simulink model "Demo_SteerableHeadlights_cs"  (Simulink 7.6)
settings: Solver=FixedStepDiscrete  SolverMode=SingleTasking  StartTime=0.0  StopTime=45  FixedStep=1/20  RelTol=1e-3
model workspace (MAT data in the model file):
  mbox_table : struct (value not decoded)
  model_closed = 0
  sim_status = 0
PreLoadFcn:
  | check_NUTS_defined;
  | 
  | assignin('base',['model_closed_' bdroot],false);
InitFcn:
  | PreScanExperimentInitFcn(bdroot)
StopFcn:
  | PreScanExperimentStopFcn(bdroot)
undefined symbols (not defined in the file or in its folder): DiscIntNeverNeededParam, x_ini_VRML, y_ini_VRML, z_ini_VRML
libraries: PreScanSimulinkLibrary x9, simulink_extras x6, simulink x4, PreScanUsefulBlocks x2
(part 1 of 4)
CloseFcn:
  | evalin('base',['clear model_closed_' bdroot]);
settings Model: Creator=PRESCAN  LastModifiedBy=buildbot
settings OptimizationCC: InitFltsAndDblsToZero=on
settings DebuggingCC: SaveWithParameterizedLinksMsg=none  SignalResolutionControl=TryResolveAllWithWarning  MultiTaskDSMMsg=warning  MultiTaskCondExecSysMsg=none
settings SFSimCC: SimParseCustomCode=off
settings RTWCC: IncludeERTFirstTime=on
settings GRTTargetCC: TargetFcnLib=ansi_tfl_tmw.mat

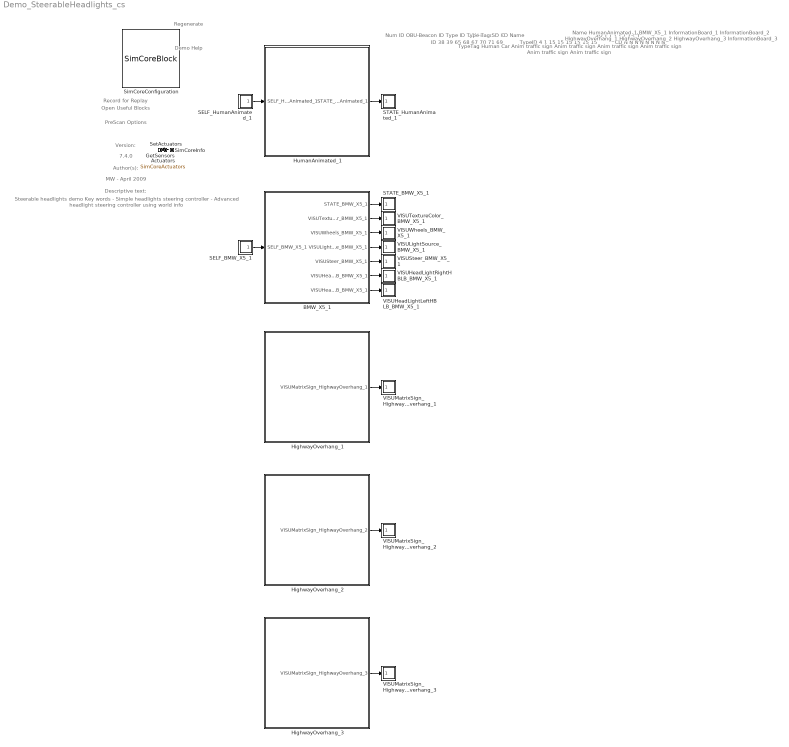
== system Demo_SteerableHeadlights_cs ==
  note: Demo Help
  note: Regenerate
  note: Record for Replay
  note: Open Useful Blocks
  note: PreScan Options
  note: Version:
  note: 7.4.0
  note: Author(s):
  note: MW - April 2009
  note: Descriptive text:
  note: Steerable headlights demo
      |
      | Key words
      | - Simple headlights steering
      | controller
      | - Advanced headlight steering
      | controller using world info
  note: ID
      |
      | 38
      | 39
      | 65
      | 68
      | 67
      | 70
      | 71
      | 69
  note: OBU-Beacon ID
  note: TypeID
      |
      | 4
      | 1
      | 15
      | 15
      | 15
      | 15
      | 15
      | 15
  note: TypeTag
      |
      | Human
      | Car
      | Anim traffic sign
      | Anim traffic sign
      | Anim traffic sign
      | Anim traffic sign
      | Anim traffic sign
      | Anim traffic sign
  note: SD
      |
      | Y
      | Y
      | Y
      | Y
      | Y
      | Y
      | Y
      | Y
  note: CD
      |
      | N
      | N
      | N
      | N
      | N
      | N
      | N
      | N
  note: Name
      |
      | HumanAnimated_1
      | BMW_X5_1
      | InformationBoard_1
      | InformationBoard_2
      | HighwayOverhang_1
      | HighwayOverhang_2
      | HighwayOverhang_3
      | InformationBoard_3
  note: Num ID OBU-Beacon ID Type ID Type Tag SD CD Name
  Actuators : DataStoreMemory  Tag=Actuators  DataStoreName=SimCoreActuators  InitialValue=zeros(288,1)
      settings: DeleteFcn=PreScanBlockDeleteFcn;
  BMW_X5_1 : Subsystem  Tag=WorldObjectSubSystem  InitFcn=UniqueId = '67';
      mask Display: image(imread('BMW_X5.jpg'));color('white');text(0,0,' ID=39\n')
  GetSensors : Subsystem  Tag=GetSensors  Priority=2  mask(PreScan Simulation Core Block){NrOfSensors=16, TimeStep=1/20}
      mask prompts: NrOfSensors "Number of sensor values"; TimeStep "Timestep [s]"
      mask help:
      | Please do not remove this block from the PreScan compilation sheet,
      | as it contains essential configuration parameters for a PreScan simulation.
      settings: DeleteFcn=PreScanBlockDeleteFcn;
  HighwayOverhang_1 : Subsystem  Tag=WorldObjectSubSystem  InitFcn=UniqueId = '104';
      mask Display: image(imread('HighwayOverhang.jpg'));color('white');text(0,0,' ID=67\n')
  HighwayOverhang_2 : Subsystem  Tag=WorldObjectSubSystem  InitFcn=UniqueId = '106';
      mask Display: image(imread('HighwayOverhang.jpg'));color('white');text(0,0,' ID=70\n')
  HighwayOverhang_3 : Subsystem  Tag=WorldObjectSubSystem  InitFcn=UniqueId = '108';
      mask Display: image(imread('HighwayOverhang.jpg'));color('white');text(0,0,' ID=71\n')
  HumanAnimated_1 : Subsystem  Tag=WorldObjectSubSystem  InitFcn=UniqueId = '63';
      mask Display: image(imread('HumanAnimated.jpg'));color('white');text(0,0,' ID=38\n')
  SELF_BMW_X5_1 : Subsystem  Tag=SELF  Priority=3  mask(PreScan Source Block: SELF){PortName=SELF_BMW_X5_1, PortIndex=8, PortWidth=8, TimeStep=1/20}
      mask prompts: PortName "Auto-Assigned: Port Name [-]"; PortIndex "Auto-Assigned: Port Index [-]"; PortWidth "Auto-Assigned: Port Dimensions"; TimeStep "Auto-Assigned: Upload Period [s]"
      mask help:
      | The SELF port shows (state) information of the actor itself. The outputs are position in the experiment's axis system and the GPS coordinates, and the object's absolute velocity and compass heading.
      |
      | For more information, please click Help.
      settings: DeleteFcn=PreScanBlockDeleteFcn;
      mask Help: eval('openHelp(462)')
      mask Display: image(imread('GPS.png'))
  SELF_HumanAnimated_1 : Subsystem  Tag=SELF  Priority=3  mask(PreScan Source Block: SELF){PortName=SELF_HumanAnimated_1, PortIndex=0, PortWidth=8, TimeStep=1/20}
      mask prompts: PortName "Auto-Assigned: Port Name [-]"; PortIndex "Auto-Assigned: Port Index [-]"; PortWidth "Auto-Assigned: Port Dimensions"; TimeStep "Auto-Assigned: Upload Period [s]"
      mask help:
      | The SELF port shows (state) information of the actor itself. The outputs are position in the experiment's axis system and the GPS coordinates, and the object's absolute velocity and compass heading.
      |
      | For more information, please click Help.
      settings: DeleteFcn=PreScanBlockDeleteFcn;
      mask Help: eval('openHelp(462)')
      mask Display: image(imread('GPS.png'))
  STATE_BMW_X5_1 : Subsystem  Tag=State  Priority=0  mask(PreScan Sink Block: State){x0=0.147277832, y0=0.07363796, z0=0.69, Roll0=0, Pitch0=0, Yaw0=0, TimeStep=1/20}
      mask prompts: x0 "Ini x-position VEHICLE wrt GLOBAL axis system [m]"; y0 "Ini y-position VEHICLE wrt GLOBAL axis system [m]"; z0 "Ini z-position VEHICLE wrt GLOBAL axis system [m]"; Roll0 "Ini roll-angle BODY wrt VEHICLE axis system [deg]"; Pitch0 "Ini pitch-angle BODY wrt VEHICLE axis system [deg]"; Yaw0 "Ini yaw-angle VEHICLE wrt GLOBAL axis system [deg]"; TimeStep "Time Step [s]"
      mask help:
      | The Actor State contains a vector signal of size (9x1), containing the following signals:
      |
      | -  Position                  (x,y,z)                                     [m]
      | -  Velocity                  (vx,vy,vz)                               [m/s]
      | -  Angles                    (Roll, Pitch, Yaw)                   [rad]
      |
      | The Actor state is defined in the global axis system.
      | The state is superponed on the Initial position defined in the GUI.
      |
      | For more information, please click Help.
      settings: DeleteFcn=PreScanBlockDeleteFcn;
      mask Help: eval('openHelp(222)')
      mask Display: image(imread('State.png'))
  STATE_HumanAnimated_1 : Subsystem  Tag=StateAnim  Priority=0  mask(PreScan Sink Block: StateAnim){x0=294.188263, y0=-30, z0=0, Roll0=0, Pitch0=0, Yaw0=102.59381900000001, TimeStep=1/20, MWS=1.95}
      mask prompts: x0 "Ini x-position VEHICLE wrt GLOBAL axis system [m]"; y0 "Ini y-position VEHICLE wrt GLOBAL axis system [m]"; z0 "Ini z-position VEHICLE wrt GLOBAL axis system [m]"; Roll0 "Ini roll-angle BODY wrt GLOBAL axis system [rad]"; Pitch0 "Ini pitch-angle BODY wrt GLOBAL axis system [rad]"; Yaw0 "Ini yaw-angle BODY wrt GLOBAL axis system [rad]"; TimeStep "Time Step [s]"; MWS "Max Walking Speed [m/s]"
      mask help:
      | The Actor State contains a vector signal of size (9x1), containing the following signals:
      |
      | -  Position                  (x,y,z)                                     [m]
      | -  Velocity                  (vx,vy,vz)                               [m/s]
      | -  Angles                    (Roll, Pitch, Yaw)                   [rad]
      |
      | The Actor state is defined in the global axis system.
      | The state is superponed on the Initial position defined in the GUI.
      |
      | For more information, please click Help.
      settings: DeleteFcn=PreScanBlockDeleteFcn;
      mask Help: eval('openHelp(222)')
      mask Display: image(imread('StateAnim.png'))
  SetActuators : Subsystem  Tag=SetActuators  Priority=1  mask(PreScan Simulation Core Block){TimeStep=1/20, NrOfActuators=288}
      mask prompts: TimeStep "Timestep [s]"; NrOfActuators "Number of actuator values"
      mask help:
      | Please do not remove this block from the PreScan compilation sheet,
      | as it contains essential configuration parameters for a PreScan simulation.
      settings: DeleteFcn=PreScanBlockDeleteFcn;
  SimCoreConfiguration : M-S-Function  Tag=SimCoreConfiguration  Description=D0CC6153B97817DA1051E6984CAAAF7B53F59DDD33C61524121AC7332DD66955  FunctionName=SimCoreBlock  Parameters=ExperimentXML PortsXML SimulationCore HostName CheckStart EnableLog RfR EnableGPUAccel ShowComputationTime  mask(PreScan Simulation Core Configurator){SimulationCore=NUTS, HostName=0, CheckStart=0, prescanversion='7.4.0', EnableLog=off, RfR=0, EnableGPUAccel=off, ShowComputationTime=off}
      mask prompts: SimulationCore "Simulation Core"; HostName "Simulation Host"; CheckStart "Show START Dialog"; prescanversion "PreScan Version"; EnableLog "Create TA Log"; RfR "Record for Replay"; EnableGPUAccel "Enable GPU Acceleration"; ShowComputationTime "Show ComputationTime Scope"
      mask help:
      | Please do not remove this block from the PreScan compilation sheet,
      | as it contains essential configuration parameter for a PreScan simulation.
      mask init:
      | model = bdroot;
      | ExperimentXML = [model(1:end-3) '.pex'];
      | PortsXML = [model '_ports.pcd'];
      settings: DeleteFcn=PreScanBlockDeleteFcn;  ModelCloseFcn=assignin('base',['model_closed_' bdroot],true);
      mask Help: eval('openHelp(812)')
      mask Display: image(imread('prescanlogo.ico'))
  SimCoreInfo : Subsystem  Tag=SimCoreInfo
  VISUHeadLightLeftHBLB_BMW_X5_1 : Subsystem  Tag=VisuLights  Priority=0
      settings: DeleteFcn=PreScanBlockDeleteFcn;
      mask Type: PreScan Sink Block: VisuLights
      mask Description:
      | The VisuLights block provides a way to animate the active lights of a vehicle with possibilities to adapt the:
      | - Intensity [-]
      | - Position (x,y,z) [m]
      | - Orientation (Roll, Pitch, Yaw) [deg]
      | - Color (RGB) [-]
      | - TextureResourceID [-]
      | 
      | For more information, please click Help.
      mask Help: eval('openHelp(231)')
      mask Display: image(imread('HeadLight.png'))
  VISUHeadLightRightHBLB_BMW_X5_1 : Subsystem  Tag=VisuLights  Priority=0
      settings: DeleteFcn=PreScanBlockDeleteFcn;
      mask Type: PreScan Sink Block: VisuLights
      mask Description:
      | The VisuLights block provides a way to animate the active lights of a vehicle with possibilities to adapt the:
      | - Intensity [-]
      | - Position (x,y,z) [m]
      | - Orientation (Roll, Pitch, Yaw) [deg]
      | - Color (RGB) [-]
      | - TextureResourceID [-]
      | 
      | For more information, please click Help.
      mask Help: eval('openHelp(231)')
      mask Display: image(imread('HeadLight.png'))
  VISULightSource_BMW_X5_1 : Subsystem  Tag=VisuLightSource  Priority=0
      settings: DeleteFcn=PreScanBlockDeleteFcn;
      mask Type: PreScan Sink Block: VisuLightSource
      mask Description:
      | The VisuLightSource block provides a way to animate Light Sources of the indicator, braking, fog and main lights of a vehicle.
      | 
      | For more information, please click Help.
      mask Help: eval('openHelp(223)')
      mask Display: image(imread('RearLight.png'))
  VISUMatrixSign_HighwayOverhang_1 : Subsystem  Tag=VisuMatrixSign  Priority=0
      settings: DeleteFcn=PreScanBlockDeleteFcn;
      mask Type: PreScan Sink Block: VisuMatrixSign
      mask Description:
      | The VisuMatrixSign block provides a way to adapt the texture of the plates connected to an overhang, based on Resource IDs of the texture files.
      | 
      | For more information, please click Help.
      mask Help: eval('openHelp()')
      mask Display: image(imread('HighwaySpeedMatrix.png'))
  VISUMatrixSign_HighwayOverhang_2 : Subsystem  Tag=VisuMatrixSign  Priority=0
      settings: DeleteFcn=PreScanBlockDeleteFcn;
      mask Type: PreScan Sink Block: VisuMatrixSign
      mask Description:
      | The VisuMatrixSign block provides a way to adapt the texture of the plates connected to an overhang, based on Resource IDs of the texture files.
      | 
      | For more information, please click Help.
      mask Help: eval('openHelp()')
      mask Display: image(imread('HighwaySpeedMatrix.png'))
  VISUMatrixSign_HighwayOverhang_3 : Subsystem  Tag=VisuMatrixSign  Priority=0
      settings: DeleteFcn=PreScanBlockDeleteFcn;
      mask Type: PreScan Sink Block: VisuMatrixSign
      mask Description:
      | The VisuMatrixSign block provides a way to adapt the texture of the plates connected to an overhang, based on Resource IDs of the texture files.
      | 
      | For more information, please click Help.
      mask Help: eval('openHelp()')
      mask Display: image(imread('HighwaySpeedMatrix.png'))
  VISUSteer_BMW_X5_1 : Subsystem  Tag=VisuSteer  Priority=0
      settings: DeleteFcn=PreScanBlockDeleteFcn;
      mask Type: PreScan Sink Block: VisuSteer
      mask Description:
      | The VisuSteer block provides a way to adapt the orientation of the steering column and steering wheel of a vehicle.
      | 
      | For more information, please click Help.
      mask Help: eval('openHelp(223)')
      mask Display: image(imread('steeringwheel.png'))
  VISUTextureColor_BMW_X5_1 : Subsystem  Tag=VisuTextureColor  Priority=0
      settings: DeleteFcn=PreScanBlockDeleteFcn;
      mask Type: PreScan Sink Block: VisuTextureColor
      mask Description:
      | The Texture Color block provides a way to adapt the color of a vehicle.
      | 
      | For more information, please click Help.
      mask Help: eval('openHelp(230)')
      mask Display: image(imread('TextureColor.png'))
  VISUWheels_BMW_X5_1 : Subsystem  Tag=VisuWheels  Priority=0
      settings: DeleteFcn=PreScanBlockDeleteFcn;
      mask Type: PreScan Sink Block: VisuWheels
      mask Description:
      | The VisuWheels block provides a way to animate the wheels of a vehicle, with steering, rotation (because of velocity) and z-displacement.
      | 
      | For more information, please click Help.
      mask Help: eval('openHelp(223)')
      mask Display: image(imread('wheel.png'))
  wires:
  HumanAnimated_1/1(STATE_HumanAnimated_1) -> STATE_HumanAnimated_1/1(State)
  SELF_HumanAnimated_1/1(U) -> HumanAnimated_1/1(SELF_HumanAnimated_1)
  BMW_X5_1/1(STATE_BMW_X5_1) -> STATE_BMW_X5_1/1(State)
  SELF_BMW_X5_1/1(U) -> BMW_X5_1/1(SELF_BMW_X5_1)
  BMW_X5_1/2(VISUTextureColor_BMW_X5_1) -> VISUTextureColor_BMW_X5_1/1(TextureColor)
  BMW_X5_1/3(VISUWheels_BMW_X5_1) -> VISUWheels_BMW_X5_1/1(Wheels)
  BMW_X5_1/4(VISULightSource_BMW_X5_1) -> VISULightSource_BMW_X5_1/1(Lights)
  BMW_X5_1/5(VISUSteer_BMW_X5_1) -> VISUSteer_BMW_X5_1/1(Steer)
  BMW_X5_1/6(VISUHeadLightRightHBLB_BMW_X5_1) -> VISUHeadLightRightHBLB_BMW_X5_1/1(Lights)
  BMW_X5_1/7(VISUHeadLightLeftHBLB_BMW_X5_1) -> VISUHeadLightLeftHBLB_BMW_X5_1/1(Lights)
  HighwayOverhang_1/1(VISUMatrixSign_HighwayOverhang_1) -> VISUMatrixSign_HighwayOverhang_1/1(MatrixSigns)
  HighwayOverhang_2/1(VISUMatrixSign_HighwayOverhang_2) -> VISUMatrixSign_HighwayOverhang_2/1(MatrixSigns)
  HighwayOverhang_3/1(VISUMatrixSign_HighwayOverhang_3) -> VISUMatrixSign_HighwayOverhang_3/1(MatrixSigns)
  SetActuators/1(dummy) -> GetSensors/1(dummy)

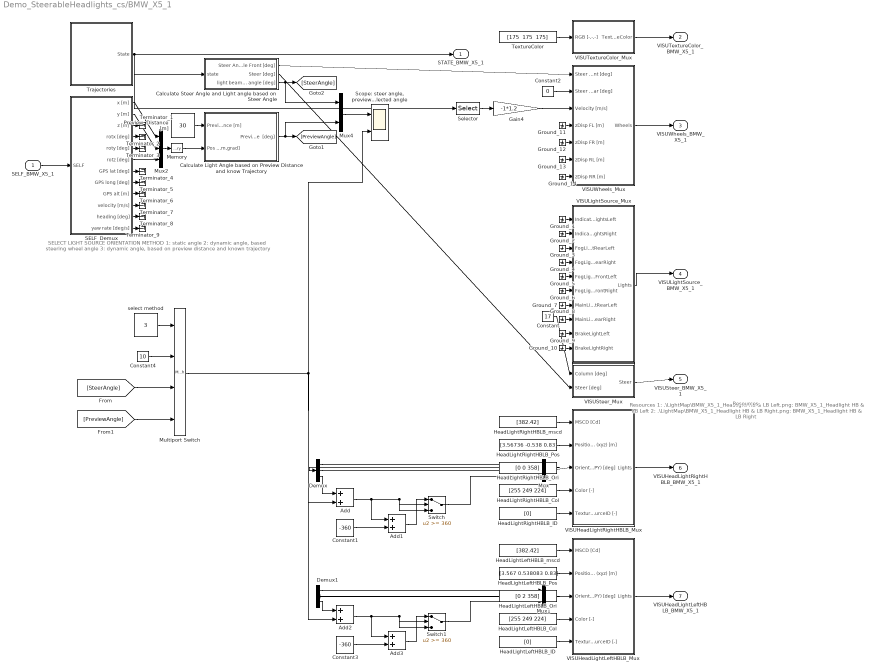
== system Demo_SteerableHeadlights_cs/BMW_X5_1 ==
  note: SELECT LIGHT SOURCE ORIENTATION METHOD
      | 1: static angle
      | 2: dynamic angle, based steering wheel angle
      | 3: dynamic angle, based on preview distance
      |     and known trajectory
  note: Resources
      |
      | 1: .\LightMap\BMW_X5_1_Headlight HB & LB Left.png: BMW_X5_1_Headlight HB & LB Left
      | 2: .\LightMap\BMW_X5_1_Headlight HB & LB Right.png: BMW_X5_1_Headlight HB & LB Right
  note: Resources
  SELF_BMW_X5_1 : Inport  Tag=SELFInport
  Add{,1..3} (4 alike) : Sum
  Calculate Light Angle based on Preview Distance and know Trajectory : Subsystem  mask{FileName=PathFollowerSva_1_Synced.mat, TrajOffset=[0 0 0]}
      mask prompts: FileName "Trajectory Name"; TrajOffset "Trajectory Initial Offset x,y,yawangle [m,m,rad]"
      mask init:
      | load(['trajectories/',FileName])
      | traject=trajectory';
      | 
      | 
      | Traj_x=(traject(:,2)*cos(TrajOffset(3))-traject(:,3)*sin(TrajOffset(3)))+TrajOffset(1);
      | Traj_y=(traject(:,2)*sin(TrajOffset(3))+traject(:,3)*cos(TrajOffset(3)))+TrajOffset(2);
  Calculate Steer Angle and Light angle based on  Steer Angle : Subsystem
  Constant : Constant  Value=17
  Constant1 : Constant  Value=-360
  Constant2 : Constant  Value=0
  Constant3 : Constant  Value=-360
  Constant4 : Constant  Value=10
  Demux : Demux  Outputs=3
  Demux1 : Demux  Outputs=3
  Gain4 : Gain  Gain=-1*1.2
  Ground_{1..14} (14 alike) : Ground
  HeadLightLeftHBLB_Col : Constant  Tag=VisuLightConst  Value=[255 249 224]
  HeadLightLeftHBLB_ID : Constant  Tag=VisuLightConst  Value=[0]
  HeadLightLeftHBLB_Ori : Constant  Tag=VisuLightConst  Value=[0 2 358]
  HeadLightLeftHBLB_Pos : Constant  Tag=VisuLightConst  Value=[3.567 0.538083 0.83]
  HeadLightLeftHBLB_mscd : Constant  Tag=VisuLightConst  Value=[382.42]
  HeadLightRightHBLB_Col : Constant  Tag=VisuLightConst  Value=[255 249 224]
  HeadLightRightHBLB_ID : Constant  Tag=VisuLightConst  Value=[0]
  HeadLightRightHBLB_Ori : Constant  Tag=VisuLightConst  Value=[0 0 358]
  HeadLightRightHBLB_Pos : Constant  Tag=VisuLightConst  Value=[3.56736 -0.538 0.83]
  HeadLightRightHBLB_mscd : Constant  Tag=VisuLightConst  Value=[382.42]
  Memory : Memory
  Multiport Switch : MultiPortSwitch  zeroidx=off
  Mux : Mux  Inputs=3
  Mux1 : Mux  Inputs=3
  Mux2 : Mux  Inputs=3
  Mux4 : Mux  Inputs=2
  Preview  Distance [m] : Constant  Value=30
  SELF_Demux : Subsystem  Tag=DemuxSELF
      settings: DeleteFcn=PreScanBlockDeleteFcn;
      mask Type: PreScan Demux Block:
      mask Display:
      | port_label('output',1,'x [m]')
      | port_label('output',2,'y [m]')
      | port_label('output',3,'z [m]','texmode','on')
      | port_label('output',4,'Rotx [deg]','texmode','on')
      | port_label('output',5,'Roty [deg]','texmode','on')
      | port_label('output',6,'Rotz [deg]','texmode','on')
      | port_label('output',7,'GPS lat [deg]','texmode','on')
      | port_label('output',8,'GPS long [deg]','texmode','on')
      | port_label('output',9,'GPS alt [m]','texmode','on')
      | port_label('output',10,'Velocity [m/s]')
      | port_label('output',11,'Heading [deg]')
      | port_label('output',12,'Yaw rate [deg/s]')
  "Scope: steer angle, preview angle, selected angle" : Scope  NumInputPorts=2
      settings: TimeRange=45  YMin=-50~-40  YMax=60~45  SaveName=ScopeData2
  Selector : Selector  InputPortWidth=9  IndexOptions=Index vector (dialog)  Indices=4  OutputSizes=1
  Switch : Switch  Threshold=360
  Switch1 : Switch  Threshold=360
  Terminator_{1..9} (9 alike) : Terminator
  TextureColor : Constant  Tag=TextureColor  Value="[175  175  175]"
  Trajectories : Subsystem  Tag=Trajectories
      settings: DeleteFcn=PreScanBlockDeleteFcn;
      mask Display: image(imread('Trajectory.png'));
  VISUHeadLightLeftHBLB_Mux : Subsystem  Tag=MuxLights
      settings: DeleteFcn=PreScanBlockDeleteFcn;
      mask Type: PreScan Mux Block:
  VISUHeadLightRightHBLB_Mux : Subsystem  Tag=MuxLights
      settings: DeleteFcn=PreScanBlockDeleteFcn;
      mask Type: PreScan Mux Block:
  VISULightSource_Mux : Subsystem  Tag=MuxLightSource
      settings: DeleteFcn=PreScanBlockDeleteFcn;
      mask Type: PreScan Mux Block:
  VISUSteer_Mux : Subsystem  Tag=MuxSteer
      settings: DeleteFcn=PreScanBlockDeleteFcn;
      mask Type: PreScan Mux Block:
  VISUTextureColor_Mux : Subsystem  Tag=MuxSteer
      settings: DeleteFcn=PreScanBlockDeleteFcn;
      mask Type: PreScan Mux Block:
  VISUWheels_Mux : Subsystem  Tag=MuxWheels  mask(PreScan Mux Block:){TimeStep=1/20}
      mask prompts: TimeStep "Auto Assigned: Time Step [s]"
      settings: DeleteFcn=PreScanBlockDeleteFcn;
  select method : Constant  Value=3
  STATE_BMW_X5_1 : Outport  Tag=StateOutport
  VISUTextureColor_BMW_X5_1 : Outport  Tag=VisuTextureColorOutport  Port=2  SampleTime=1/20
  VISUWheels_BMW_X5_1 : Outport  Tag=VisuWheelsOutport  Port=3  SampleTime=1/20
  VISULightSource_BMW_X5_1 : Outport  Tag=VisuLightsOutport  Port=4  SampleTime=1/20
  VISUSteer_BMW_X5_1 : Outport  Tag=VisuSteerOutport  Port=5  SampleTime=1/20
  VISUHeadLightRightHBLB_BMW_X5_1 : Outport  Tag=VisuHeadLightRightHBLBOutport  Port=6  SampleTime=1/20
  VISUHeadLightLeftHBLB_BMW_X5_1 : Outport  Tag=VisuHeadLightLeftHBLBOutport  Port=7  SampleTime=1/20
  wires:
  Preview  Distance [m]/1 -> Calculate Light Angle based on Preview Distance and know Trajectory/1(Preview Distance [m])
  Mux2/1 -> Memory/1
  Selector/1 -> Gain4/1
  [PreviewAngle] -> Multiport Switch/4
  Constant4/1 -> Multiport Switch/2
  select method/1 -> Multiport Switch/1
  Multiport Switch/1 -> "Scope: steer angle, preview angle, selected angle"/2, Add/2, Add2/2
  Mux4/1 -> "Scope: steer angle, preview angle, selected angle"/1
  Memory/1 -> Calculate Light Angle based on Preview Distance and know Trajectory/2(Pos x,y,Y [m,m,grad])
  Calculate Steer Angle and Light angle based on  Steer Angle/3(light beam angle [deg]) -> [SteerAngle], Mux4/1
  Calculate Light Angle based on Preview Distance and know Trajectory/1(PreviewAngle  [deg]) -> [PreviewAngle], Mux4/2
  [SteerAngle] -> Multiport Switch/3
  Demux/1 -> Mux/1
  Demux/2 -> Mux/2
  Demux/3 -> Add/1
  Switch/1 -> Mux/3
  Demux1/1 -> Mux1/1
  Demux1/2 -> Mux1/2
  Add/1 -> Add1/1, Switch/2, Switch/3
  Constant1/1 -> Add1/2
  Add1/1 -> Switch/1
  Add2/1 -> Add3/1, Switch1/2, Switch1/3
  Constant3/1 -> Add3/2
  Add3/1 -> Switch1/1
  Demux1/3 -> Add2/1
  Switch1/1 -> Mux1/3
  SELF_BMW_X5_1/1 -> SELF_Demux/1(SELF)
  VISUTextureColor_Mux/1(TextureColor) -> VISUTextureColor_BMW_X5_1/1
  TextureColor/1 -> VISUTextureColor_Mux/1(RGB [-,-,-])
  VISUWheels_Mux/1(Wheels) -> VISUWheels_BMW_X5_1/1
  VISULightSource_Mux/1(Lights) -> VISULightSource_BMW_X5_1/1
  VISUSteer_Mux/1(Steer) -> VISUSteer_BMW_X5_1/1
  VISUHeadLightRightHBLB_Mux/1(Lights) -> VISUHeadLightRightHBLB_BMW_X5_1/1
  HeadLightRightHBLB_mscd/1 -> VISUHeadLightRightHBLB_Mux/1(MSCD [Cd])
  HeadLightRightHBLB_Pos/1 -> VISUHeadLightRightHBLB_Mux/2(Position (xyz) [m])
  HeadLightRightHBLB_Ori/1 -> Demux/1
  HeadLightRightHBLB_Col/1 -> VISUHeadLightRightHBLB_Mux/4(Color [-])
  HeadLightRightHBLB_ID/1 -> VISUHeadLightRightHBLB_Mux/5(TextureResourceID [-])
  VISUHeadLightLeftHBLB_Mux/1(Lights) -> VISUHeadLightLeftHBLB_BMW_X5_1/1
  HeadLightLeftHBLB_mscd/1 -> VISUHeadLightLeftHBLB_Mux/1(MSCD [Cd])
  HeadLightLeftHBLB_Pos/1 -> VISUHeadLightLeftHBLB_Mux/2(Position (xyz) [m])
  HeadLightLeftHBLB_Col/1 -> VISUHeadLightLeftHBLB_Mux/4(Color [-])
  HeadLightLeftHBLB_ID/1 -> VISUHeadLightLeftHBLB_Mux/5(TextureResourceID [-])
  Trajectories/1(State) -> STATE_BMW_X5_1/1, Calculate Steer Angle and Light angle based on  Steer Angle/1(state), Selector/1
  Calculate Steer Angle and Light angle based on  Steer Angle/2(Steer [deg]) -> VISUSteer_Mux/2(Steer [deg])
  Gain4/1 -> VISUWheels_Mux/3(Velocity [m/s])
  Constant2/1 -> VISUWheels_Mux/2(Steer Angle Rear [deg])
  Calculate Steer Angle and Light angle based on  Steer Angle/1(Steer Angle Front [deg]) -> VISUWheels_Mux/1(Steer Angle Front [deg])
  Constant/1 -> VISUSteer_Mux/1(Column [deg])
  SELF_Demux/6(rotz [deg]) -> Mux2/3
  SELF_Demux/2(y [m]) -> Mux2/2
  SELF_Demux/1(x [m]) -> Mux2/1
  Mux/1 -> VISUHeadLightRightHBLB_Mux/3(Orientation (RPY) [deg])
  Mux1/1 -> VISUHeadLightLeftHBLB_Mux/3(Orientation (RPY) [deg])
  HeadLightLeftHBLB_Ori/1 -> Demux1/1
  SELF_Demux/3(z [m]) -> Terminator_1/1
  SELF_Demux/4(rotx [deg]) -> Terminator_2/1
  SELF_Demux/5(roty [deg]) -> Terminator_3/1
  SELF_Demux/7(GPS lat [deg]) -> Terminator_4/1
  SELF_Demux/8(GPS long [deg]) -> Terminator_5/1
  SELF_Demux/9(GPS alt [m]) -> Terminator_6/1
  SELF_Demux/10(velocity [m/s]) -> Terminator_7/1
  SELF_Demux/11(heading [deg]) -> Terminator_8/1
  SELF_Demux/12(yaw rate [deg/s]) -> Terminator_9/1
  Ground_1/1 -> VISULightSource_Mux/1(IndicatorLightsLeft)
  Ground_2/1 -> VISULightSource_Mux/2(IndicatorLightsRight)
  Ground_3/1 -> VISULightSource_Mux/3(FogLightRearLeft)
  Ground_4/1 -> VISULightSource_Mux/4(FogLightRearRight)
  Ground_5/1 -> VISULightSource_Mux/5(FogLightFrontLeft)
  Ground_6/1 -> VISULightSource_Mux/6(FogLightFrontRight)
  Ground_7/1 -> VISULightSource_Mux/7(MainLightRearLeft)
  Ground_8/1 -> VISULightSource_Mux/8(MainLightRearRight)
  Ground_9/1 -> VISULightSource_Mux/9(BrakeLightLeft)
  Ground_10/1 -> VISULightSource_Mux/10(BrakeLightRight)
  Ground_11/1 -> VISUWheels_Mux/4(zDisp FL [m])
  Ground_12/1 -> VISUWheels_Mux/5(zDisp FR [m])
  Ground_13/1 -> VISUWheels_Mux/6(zDisp RL [m])
  Ground_14/1 -> VISUWheels_Mux/7(zDisp RR [m])

== system Demo_SteerableHeadlights_cs/GetSensors ==
  dummy : Inport
  GetSensors : M-S-Function  FunctionName=GetSensorsBlock  Parameters=TimeStep NrOfSensors
  tag scope: SimCoreSensors=global
  wires:
  GetSensors/1 -> [SimCoreSensors]
  dummy/1 -> GetSensors/1

== system Demo_SteerableHeadlights_cs/HighwayOverhang_1 ==
  note: Resources
      |
      | 2: .\InformationSign\Tno.png: Tno
      | 3: InformationSign\SmallPreScan.bmp: SmallPreScan
  note: Resources
  Ground_1 : Ground
  VISUMatrixSign_Mux : Subsystem  Tag=MuxMatrixSign
      settings: DeleteFcn=PreScanBlockDeleteFcn;
      mask Type: PreScan Mux Block:
  VISUMatrixSign_HighwayOverhang_1 : Outport  Tag=VisuMatrixSignOutport  SampleTime=1/20
  wires:
  VISUMatrixSign_Mux/1(MatrixSigns) -> VISUMatrixSign_HighwayOverhang_1/1
  Ground_1/1 -> VISUMatrixSign_Mux/1(InformationPlate_1)

== system Demo_SteerableHeadlights_cs/HighwayOverhang_2 ==
  note: Resources
      |
      | 2: .\InformationSign\Tno.png: Tno
      | 3: InformationSign\SmallPreScan.bmp: SmallPreScan
  note: Resources
  Ground_1 : Ground
  VISUMatrixSign_Mux : Subsystem  Tag=MuxMatrixSign
      settings: DeleteFcn=PreScanBlockDeleteFcn;
      mask Type: PreScan Mux Block:
  VISUMatrixSign_HighwayOverhang_2 : Outport  Tag=VisuMatrixSignOutport  SampleTime=1/20
  wires:
  VISUMatrixSign_Mux/1(MatrixSigns) -> VISUMatrixSign_HighwayOverhang_2/1
  Ground_1/1 -> VISUMatrixSign_Mux/1(InformationPlate_2)

== system Demo_SteerableHeadlights_cs/HighwayOverhang_3 ==
  note: Resources
      |
      | 2: .\InformationSign\Tno.png: Tno
      | 3: InformationSign\SmallPreScan.bmp: SmallPreScan
  note: Resources
  Ground_1 : Ground
  VISUMatrixSign_Mux : Subsystem  Tag=MuxMatrixSign
      settings: DeleteFcn=PreScanBlockDeleteFcn;
      mask Type: PreScan Mux Block:
  VISUMatrixSign_HighwayOverhang_3 : Outport  Tag=VisuMatrixSignOutport  SampleTime=1/20
  wires:
  VISUMatrixSign_Mux/1(MatrixSigns) -> VISUMatrixSign_HighwayOverhang_3/1
  Ground_1/1 -> VISUMatrixSign_Mux/1(InformationPlate_3)

== system Demo_SteerableHeadlights_cs/HumanAnimated_1 ==
  SELF_HumanAnimated_1 : Inport  Tag=SELFInport
  SELF_Demux : Subsystem  Tag=DemuxSELF
      settings: DeleteFcn=PreScanBlockDeleteFcn;
      mask Type: PreScan Demux Block:
      mask Display:
      | port_label('output',1,'x [m]')
      | port_label('output',2,'y [m]')
      | port_label('output',3,'z [m]','texmode','on')
      | port_label('output',4,'Rotx [deg]','texmode','on')
      | port_label('output',5,'Roty [deg]','texmode','on')
      | port_label('output',6,'Rotz [deg]','texmode','on')
      | port_label('output',7,'GPS lat [deg]','texmode','on')
      | port_label('output',8,'GPS long [deg]','texmode','on')
      | port_label('output',9,'GPS alt [m]','texmode','on')
      | port_label('output',10,'Velocity [m/s]')
      | port_label('output',11,'Heading [deg]')
      | port_label('output',12,'Yaw rate [deg/s]')
  Terminator_{1..12} (12 alike) : Terminator
  Trajectories : Subsystem  Tag=Trajectories
      settings: DeleteFcn=PreScanBlockDeleteFcn;
      mask Display: image(imread('Trajectory.png'));
  STATE_HumanAnimated_1 : Outport  Tag=StateOutport
  wires:
  SELF_HumanAnimated_1/1 -> SELF_Demux/1(SELF)
  Trajectories/1(State) -> STATE_HumanAnimated_1/1
  SELF_Demux/1(x [m]) -> Terminator_1/1
  SELF_Demux/2(y [m]) -> Terminator_2/1
  SELF_Demux/3(z [m]) -> Terminator_3/1
  SELF_Demux/4(rotx [deg]) -> Terminator_4/1
  SELF_Demux/5(roty [deg]) -> Terminator_5/1
  SELF_Demux/6(rotz [deg]) -> Terminator_6/1
  SELF_Demux/7(GPS lat [deg]) -> Terminator_7/1
  SELF_Demux/8(GPS long [deg]) -> Terminator_8/1
  SELF_Demux/9(GPS alt [m]) -> Terminator_9/1
  SELF_Demux/10(velocity [m/s]) -> Terminator_10/1
  SELF_Demux/11(heading [deg]) -> Terminator_11/1
  SELF_Demux/12(yaw rate [deg/s]) -> Terminator_12/1

== system Demo_SteerableHeadlights_cs/SELF_BMW_X5_1 ==
  Selector : Selector  IndexMode=Zero-based  IndexOptions=Starting index (dialog)  Indices=PortIndex  OutputSizes=PortWidth(1)
  U : Outport
  wires:
  Selector/1 -> U/1
  [SimCoreSensors] -> Selector/1

== system Demo_SteerableHeadlights_cs/SELF_HumanAnimated_1 ==
  Selector : Selector  IndexMode=Zero-based  IndexOptions=Starting index (dialog)  Indices=PortIndex  OutputSizes=PortWidth(1)
  U : Outport
  wires:
  Selector/1 -> U/1
  [SimCoreSensors] -> Selector/1

== system Demo_SteerableHeadlights_cs/STATE_BMW_X5_1 ==
  State : Inport  SampleTime=TimeStep
  Acceleration : Subsystem  mask(ToSensorWorld){PortName=Acceleration_BMW_X5_1, PortIndex=23, PortWidth=3, TimeStep=1/20}
      mask prompts: PortName "Port Name [-]"; PortIndex "Index [-]"; PortWidth "Port Dimensions [-]"; TimeStep "Upload Period [s]"
      mask help: Sends signal(s) from Simulink to the Sensor World
      mask Help:
      | Sends signal(s) from Simulink to the Sensor World.
      | 
      | - Port Name [-]: specifies the name of the output terminal of the Simulink block.
      | - Index [-]: specifies the start position in the output vector sent to the Sensor World
      | - Port dimensions [-]: specifies the width (number of scalars) of the output port
      | - Upload period [s]: specifies the upload period (in seconds) of the port.
      mask Display: port_label('input', 1, PortName)
  Demux : Demux  Outputs=5
  Position : Subsystem  mask(ToSensorWorld){PortName=Position_BMW_X5_1, PortIndex=17, PortWidth=3, TimeStep=1/20}
      mask prompts: PortName "Port Name [-]"; PortIndex "Index [-]"; PortWidth "Port Dimensions [-]"; TimeStep "Upload Period [s]"
      mask help: Sends signal(s) from Simulink to the Sensor World
      mask Help:
      | Sends signal(s) from Simulink to the Sensor World.
      | 
      | - Port Name [-]: specifies the name of the output terminal of the Simulink block.
      | - Index [-]: specifies the start position in the output vector sent to the Sensor World
      | - Port dimensions [-]: specifies the width (number of scalars) of the output port
      | - Upload period [s]: specifies the upload period (in seconds) of the port.
      mask Display: port_label('input', 1, PortName)
  RPY : Subsystem  mask(ToSensorWorld){PortName=RPY_BMW_X5_1, PortIndex=26, PortWidth=3, TimeStep=1/20}
      mask prompts: PortName "Port Name [-]"; PortIndex "Index [-]"; PortWidth "Port Dimensions [-]"; TimeStep "Upload Period [s]"
      mask help: Sends signal(s) from Simulink to the Sensor World
      mask Help:
      | Sends signal(s) from Simulink to the Sensor World.
      | 
      | - Port Name [-]: specifies the name of the output terminal of the Simulink block.
      | - Index [-]: specifies the start position in the output vector sent to the Sensor World
      | - Port dimensions [-]: specifies the width (number of scalars) of the output port
      | - Upload period [s]: specifies the upload period (in seconds) of the port.
      mask Display: port_label('input', 1, PortName)
  Velocity : Subsystem  mask(ToSensorWorld){PortName=Velocity_BMW_X5_1, PortIndex=20, PortWidth=3, TimeStep=1/20}
      mask prompts: PortName "Port Name [-]"; PortIndex "Index [-]"; PortWidth "Port Dimensions [-]"; TimeStep "Upload Period [s]"
      mask help: Sends signal(s) from Simulink to the Sensor World
      mask Help:
      | Sends signal(s) from Simulink to the Sensor World.
      | 
      | - Port Name [-]: specifies the name of the output terminal of the Simulink block.
      | - Index [-]: specifies the start position in the output vector sent to the Sensor World
      | - Port dimensions [-]: specifies the width (number of scalars) of the output port
      | - Upload period [s]: specifies the upload period (in seconds) of the port.
      mask Display: port_label('input', 1, PortName)
  iniBODYAngles wrtVEH [rad] : Constant  Value=[Roll0 Pitch0 0]  SampleTime=TimeStep
  iniVEHAngles wrtGLOB [rad] : Constant  Value=[0 0 Yaw0]  SampleTime=TimeStep
  iniVEHposition wrtGLOB [m] : Constant  Value=[x0 y0 z0]  SampleTime=TimeStep
  state2FullState : PreScanSimulinkLibrary/state2FullState  SystemSampleTime=-1
  velRPY : Subsystem  mask(ToSensorWorld){PortName=velRPY_BMW_X5_1, PortIndex=29, PortWidth=3, TimeStep=1/20}
      mask prompts: PortName "Port Name [-]"; PortIndex "Index [-]"; PortWidth "Port Dimensions [-]"; TimeStep "Upload Period [s]"
      mask help: Sends signal(s) from Simulink to the Sensor World
      mask Help:
      | Sends signal(s) from Simulink to the Sensor World.
      | 
      | - Port Name [-]: specifies the name of the output terminal of the Simulink block.
      | - Index [-]: specifies the start position in the output vector sent to the Sensor World
      | - Port dimensions [-]: specifies the width (number of scalars) of the output port
      | - Upload period [s]: specifies the upload period (in seconds) of the port.
      mask Display: port_label('input', 1, PortName)
  wires:
  Demux/5 -> velRPY/1(Y)
  Demux/4 -> RPY/1(Y)
  Demux/3 -> Acceleration/1(Y)
  Demux/2 -> Velocity/1(Y)
  Demux/1 -> Position/1(Y)
  State/1 -> state2FullState/1
  state2FullState/1 -> Demux/1
  iniVEHposition wrtGLOB [m]/1 -> state2FullState/2
  iniBODYAngles wrtVEH [rad]/1 -> state2FullState/3
  iniVEHAngles wrtGLOB [rad]/1 -> state2FullState/4

== system Demo_SteerableHeadlights_cs/STATE_HumanAnimated_1 ==
  State : Inport  SampleTime=TimeStep
  Acceleration : Subsystem  mask(ToSensorWorld){PortName=Acceleration_HumanAnimated_1, PortIndex=6, PortWidth=3, TimeStep=1/20}
      mask prompts: PortName "Port Name [-]"; PortIndex "Index [-]"; PortWidth "Port Dimensions [-]"; TimeStep "Upload Period [s]"
      mask help: Sends signal(s) from Simulink to the Sensor World
      mask Help:
      | Sends signal(s) from Simulink to the Sensor World.
      | 
      | - Port Name [-]: specifies the name of the output terminal of the Simulink block.
      | - Index [-]: specifies the start position in the output vector sent to the Sensor World
      | - Port dimensions [-]: specifies the width (number of scalars) of the output port
      | - Upload period [s]: specifies the upload period (in seconds) of the port.
      mask Display: port_label('input', 1, PortName)
  Anim : Subsystem  mask(ToSensorWorld){PortName=Anim_HumanAnimated_1, PortIndex=15, PortWidth=2, TimeStep=1/20}
      mask prompts: PortName "Port Name [-]"; PortIndex "Index [-]"; PortWidth "Port Dimensions [-]"; TimeStep "Upload Period [s]"
      mask help: Sends signal(s) from Simulink to the Sensor World
      mask Help:
      | Sends signal(s) from Simulink to the Sensor World.
      | 
      | - Port Name [-]: specifies the name of the output terminal of the Simulink block.
      | - Index [-]: specifies the start position in the output vector sent to the Sensor World
      | - Port dimensions [-]: specifies the width (number of scalars) of the output port
      | - Upload period [s]: specifies the upload period (in seconds) of the port.
      mask Display: port_label('input', 1, PortName)
  Demux : Demux  Outputs=5
  Mux : Mux  Inputs=2
  Position : Subsystem  mask(ToSensorWorld){PortName=Position_HumanAnimated_1, PortIndex=0, PortWidth=3, TimeStep=1/20}
      mask prompts: PortName "Port Name [-]"; PortIndex "Index [-]"; PortWidth "Port Dimensions [-]"; TimeStep "Upload Period [s]"
      mask help: Sends signal(s) from Simulink to the Sensor World
      mask Help:
      | Sends signal(s) from Simulink to the Sensor World.
      | 
      | - Port Name [-]: specifies the name of the output terminal of the Simulink block.
      | - Index [-]: specifies the start position in the output vector sent to the Sensor World
      | - Port dimensions [-]: specifies the width (number of scalars) of the output port
      | - Upload period [s]: specifies the upload period (in seconds) of the port.
      mask Display: port_label('input', 1, PortName)
  RPY : Subsystem  mask(ToSensorWorld){PortName=RPY_HumanAnimated_1, PortIndex=9, PortWidth=3, TimeStep=1/20}
      mask prompts: PortName "Port Name [-]"; PortIndex "Index [-]"; PortWidth "Port Dimensions [-]"; TimeStep "Upload Period [s]"
      mask help: Sends signal(s) from Simulink to the Sensor World
      mask Help:
      | Sends signal(s) from Simulink to the Sensor World.
      | 
      | - Port Name [-]: specifies the name of the output terminal of the Simulink block.
      | - Index [-]: specifies the start position in the output vector sent to the Sensor World
      | - Port dimensions [-]: specifies the width (number of scalars) of the output port
      | - Upload period [s]: specifies the upload period (in seconds) of the port.
      mask Display: port_label('input', 1, PortName)
  Velocity : Subsystem  mask(ToSensorWorld){PortName=Velocity_HumanAnimated_1, PortIndex=3, PortWidth=3, TimeStep=1/20}
      mask prompts: PortName "Port Name [-]"; PortIndex "Index [-]"; PortWidth "Port Dimensions [-]"; TimeStep "Upload Period [s]"
      mask help: Sends signal(s) from Simulink to the Sensor World
      mask Help:
      | Sends signal(s) from Simulink to the Sensor World.
      | 
      | - Port Name [-]: specifies the name of the output terminal of the Simulink block.
      | - Index [-]: specifies the start position in the output vector sent to the Sensor World
      | - Port dimensions [-]: specifies the width (number of scalars) of the output port
      | - Upload period [s]: specifies the upload period (in seconds) of the port.
      mask Display: port_label('input', 1, PortName)
  animation mode : Subsystem
  elapsed track : PreScanSimulinkLibrary/StateAnimC/elapsed track  SystemSampleTime=-1
  iniBODYAngles wrtVEH [rad] : Constant  Value=[Roll0 Pitch0 0]  SampleTime=TimeStep
  iniVEHAngles wrtGLOB [rad] : Constant  Value=[0 0 Yaw0]  SampleTime=TimeStep
  iniVEHposition wrtGLOB [m] : Constant  Value=[x0 y0 z0]  SampleTime=TimeStep
  state2FullState : PreScanSimulinkLibrary/state2FullState  SystemSampleTime=-1
  velRPY : Subsystem  mask(ToSensorWorld){PortName=velRPY_HumanAnimated_1, PortIndex=12, PortWidth=3, TimeStep=1/20}
      mask prompts: PortName "Port Name [-]"; PortIndex "Index [-]"; PortWidth "Port Dimensions [-]"; TimeStep "Upload Period [s]"
      mask help: Sends signal(s) from Simulink to the Sensor World
      mask Help:
      | Sends signal(s) from Simulink to the Sensor World.
      | 
      | - Port Name [-]: specifies the name of the output terminal of the Simulink block.
      | - Index [-]: specifies the start position in the output vector sent to the Sensor World
      | - Port dimensions [-]: specifies the width (number of scalars) of the output port
      | - Upload period [s]: specifies the upload period (in seconds) of the port.
      mask Display: port_label('input', 1, PortName)
  wires:
  State/1 -> state2FullState/1
  iniVEHAngles wrtGLOB [rad]/1 -> state2FullState/4
  iniBODYAngles wrtVEH [rad]/1 -> state2FullState/3
  iniVEHposition wrtGLOB [m]/1 -> state2FullState/2
  state2FullState/1 -> Demux/1
  Demux/5 -> velRPY/1(Y)
  Demux/4 -> RPY/1(Y)
  Demux/3 -> Acceleration/1(Y)
  Demux/2 -> elapsed track/1, animation mode/1(vel), Velocity/1(Y)
  Demux/1 -> Position/1(Y)
  Mux/1 -> Anim/1(Y)
  animation mode/1(mode) -> Mux/1
  elapsed track/1 -> Mux/2

== system Demo_SteerableHeadlights_cs/SetActuators ==
  Bus Creator : BusCreator  Inputs=1
  Data Store Read : DataStoreRead  DataStoreName=SimCoreActuators  SampleTime=TimeStep
  SendActuators : M-S-Function  FunctionName=SendActuatorsBlock  Parameters=TimeStep NrOfActuators
  dummy : Outport
  tag scope: SimCoreInfo=global
  wires:
  Bus Creator/1 -> [SimCoreInfo]  "SimCore"
  SendActuators/2 -> Bus Creator/1  "ComputationTime[s]"
  SendActuators/1 -> dummy/1
  Data Store Read/1 -> SendActuators/1

== system Demo_SteerableHeadlights_cs/SimCoreInfo ==
  Bus Selector : BusSelector  OutputSignals=ComputationTime[s]
  Time : Scope
      settings: TimeRange=10  YMin=0  YMax=0.5  SaveName=ComputationTime
  wires:
  Bus Selector/1 -> Time/1  "<ComputationTime[s]>"
  [SimCoreInfo] -> Bus Selector/1

== system Demo_SteerableHeadlights_cs/VISUHeadLightLeftHBLB_BMW_X5_1 ==
  Lights : Inport
  Bus Selector : BusSelector  OutputSignals=Intensity,Position,Orientation,Color,TextureResourceID
  Compare To Zero : simulink/Logic and Bit Operations/Compare To Zero  SystemSampleTime=-1  relop=~=  LogicOutDataTypeMode=uint8  ZeroCross=off
  Data Type Conversion : DataTypeConversion  OutDataTypeStr=double
  Degrees to Radians : simulink_extras/Transformations/Degrees to Radians  SystemSampleTime=-1
  HDR scale calculation : Subsystem
  Mux : Mux  Inputs=2
  ambient diffuse specular : Selector  InputPortWidth=16  IndexOptions=Index vector (dialog)  Indices=[1:12]  OutputSizes=12
  conv_MeshColor : Subsystem
  emission RGBA : Selector  InputPortWidth=16  IndexOptions=Index vector (dialog)  Indices=[13:16]  OutputSizes=3
  scaler : Subsystem
  visu_ColorLight : Subsystem  mask(ToSensorWorld){PortName=visu_DynLightVehicleHeadLightLeftHBLBColor_0, PortIndex=265, PortWidth=3, TimeStep=1/20}
      mask prompts: PortName "Port Name [-]"; PortIndex "Index [-]"; PortWidth "Port Dimensions [-]"; TimeStep "Upload Period [s]"
      mask help: Sends signal(s) from Simulink to the Sensor World
      mask Help:
      | Sends signal(s) from Simulink to the Sensor World.
      | 
      | - Port Name [-]: specifies the name of the output terminal of the Simulink block.
      | - Index [-]: specifies the start position in the output vector sent to the Sensor World
      | - Port dimensions [-]: specifies the width (number of scalars) of the output port
      | - Upload period [s]: specifies the upload period (in seconds) of the port.
      mask Display: port_label('input', 1, PortName)
  visu_ICMLight : Subsystem  mask(ToSensorWorld){PortName=visu_DynLightVehicleHeadLightLeftHBLBICM_0, PortIndex=284, PortWidth=1, TimeStep=1/20}
      mask prompts: PortName "Port Name [-]"; PortIndex "Index [-]"; PortWidth "Port Dimensions [-]"; TimeStep "Upload Period [s]"
      mask help: Sends signal(s) from Simulink to the Sensor World
      mask Help:
      | Sends signal(s) from Simulink to the Sensor World.
      | 
      | - Port Name [-]: specifies the name of the output terminal of the Simulink block.
      | - Index [-]: specifies the start position in the output vector sent to the Sensor World
      | - Port dimensions [-]: specifies the width (number of scalars) of the output port
      | - Upload period [s]: specifies the upload period (in seconds) of the port.
      mask Display: port_label('input', 1, PortName)
  visu_IntLight : Subsystem  mask(ToSensorWorld){PortName=visu_DynLightVehicleHeadLightLeftHBLB_0, PortIndex=258, PortWidth=1, TimeStep=1/20}
      mask prompts: PortName "Port Name [-]"; PortIndex "Index [-]"; PortWidth "Port Dimensions [-]"; TimeStep "Upload Period [s]"
      mask help: Sends signal(s) from Simulink to the Sensor World
      mask Help:
      | Sends signal(s) from Simulink to the Sensor World.
      | 
      | - Port Name [-]: specifies the name of the output terminal of the Simulink block.
      | - Index [-]: specifies the start position in the output vector sent to the Sensor World
      | - Port dimensions [-]: specifies the width (number of scalars) of the output port
      | - Upload period [s]: specifies the upload period (in seconds) of the port.
      mask Display: port_label('input', 1, PortName)
  visu_MeshLight : Subsystem  mask(ToSensorWorld){PortName=visu_MainLightFrontLeft_0, PortIndex=268, PortWidth=16, TimeStep=1/20}
      mask prompts: PortName "Port Name [-]"; PortIndex "Index [-]"; PortWidth "Port Dimensions [-]"; TimeStep "Upload Period [s]"
      mask help: Sends signal(s) from Simulink to the Sensor World
      mask Help:
      | Sends signal(s) from Simulink to the Sensor World.
      | 
      | - Port Name [-]: specifies the name of the output terminal of the Simulink block.
      | - Index [-]: specifies the start position in the output vector sent to the Sensor World
      | - Port dimensions [-]: specifies the width (number of scalars) of the output port
      | - Upload period [s]: specifies the upload period (in seconds) of the port.
      mask Display: port_label('input', 1, PortName)
  visu_RotLight : Subsystem  mask(ToSensorWorld){PortName=visu_DynLightVehicleHeadLightLeftHBLBRot_0, PortIndex=262, PortWidth=3, TimeStep=1/20}
      mask prompts: PortName "Port Name [-]"; PortIndex "Index [-]"; PortWidth "Port Dimensions [-]"; TimeStep "Upload Period [s]"
      mask help: Sends signal(s) from Simulink to the Sensor World
      mask Help:
      | Sends signal(s) from Simulink to the Sensor World.
      | 
      | - Port Name [-]: specifies the name of the output terminal of the Simulink block.
      | - Index [-]: specifies the start position in the output vector sent to the Sensor World
      | - Port dimensions [-]: specifies the width (number of scalars) of the output port
      | - Upload period [s]: specifies the upload period (in seconds) of the port.
      mask Display: port_label('input', 1, PortName)
  visu_TransLight : Subsystem  mask(ToSensorWorld){PortName=visu_DynLightVehicleHeadLightLeftHBLBTrans_0, PortIndex=259, PortWidth=3, TimeStep=1/20}
      mask prompts: PortName "Port Name [-]"; PortIndex "Index [-]"; PortWidth "Port Dimensions [-]"; TimeStep "Upload Period [s]"
      mask help: Sends signal(s) from Simulink to the Sensor World
      mask Help:
      | Sends signal(s) from Simulink to the Sensor World.
      | 
      | - Port Name [-]: specifies the name of the output terminal of the Simulink block.
      | - Index [-]: specifies the start position in the output vector sent to the Sensor World
      | - Port dimensions [-]: specifies the width (number of scalars) of the output port
      | - Upload period [s]: specifies the upload period (in seconds) of the port.
      mask Display: port_label('input', 1, PortName)
  wires:
  emission RGBA/1 -> scaler/1(RGBA)
  scaler/1(scaled RGBA) -> Mux/2
  Mux/1 -> visu_MeshLight/1(Y)
  ambient diffuse specular/1 -> Mux/1
  conv_MeshColor/1(RGBcolor) -> emission RGBA/1, ambient diffuse specular/1
  HDR scale calculation/1(Emission Scale) -> scaler/2(Scale)
  Bus Selector/5 -> visu_ICMLight/1(Y)  "<TextureResourceID>"
  Data Type Conversion/1 -> conv_MeshColor/1(on_off)
  Compare To Zero/1 -> Data Type Conversion/1
  Bus Selector/4 -> visu_ColorLight/1(Y)  "<Color>"
  Bus Selector/3 -> Degrees to Radians/1  "<Orientation>"
  Bus Selector/2 -> visu_TransLight/1(Y)  "<Position>"
  Degrees to Radians/1 -> visu_RotLight/1(Y)
  Lights/1 -> Bus Selector/1
  Bus Selector/1 -> HDR scale calculation/1(Intensity), visu_IntLight/1(Y), Compare To Zero/1  "<Intensity>"
